simulink model "l17_ex1_LC"  (R2018b)
settings: Solver=ode45  StartTime=0.0  StopTime=5  MaxStep=1e-5  RelTol=1e-4  AbsTol=1e-4  EnableMultiTasking=on
values from neighbouring files (symbols this model uses):
  K = 1    [l16.m]    (also in l17.m = 5.3)
  p1 = 2.65    [l17.m]
  z1 = 1    [l17.m]
settings Model: Creator=Joe  LastModifiedBy=joema
settings SolverCC: AutoScaleAbsTol=off
settings DataIOCC: LimitDataPoints=on  SaveFormat=Array
settings OptimizationCC: LifeSpan=inf
settings DebuggingCC: UnderspecifiedInitializationDetection=Classic  MergeDetectMultiDrivingBlocksExec=none  LibraryContextMissingDiagnostic=none  SFUnexpectedBacktrackingDiag=warning  SFNoUnconditionalDefaultTransitionDiag=warning  SFExecutionAtInitializationDiag=none
settings HardwareCC: ProdBitPerPointer=32  ProdBitPerSizeT=32  ProdBitPerPtrDiffT=32  ProdLargestAtomicFloat=None  ProdIntDivRoundTo=Undefined  ProdEndianess=Unspecified  ProdWordSize=32  ProdHWDeviceType=32-bit Generic
settings ModelReferenceCC: PropagateSignalLabelsOutOfModel=off
settings SFSimCC: SimUseLocalCustomCode=off
settings RTWCC: RTWUseLocalCustomCode=off
settings CodeAppCC: StateflowObjectComments=on
settings GRTTargetCC: TargetLangStandard=C89/C90 (ANSI)  GeneratePreprocessorConditionals=Disable all
settings ConfigComp: CovMetricSettings=dw  CovHtmlReporting=on  CovSaveCumulativeToWorkspaceVar=on  CovSaveSingleToWorkspaceVar=on  CovExternalEMLEnable=off  CovSFcnEnable=off

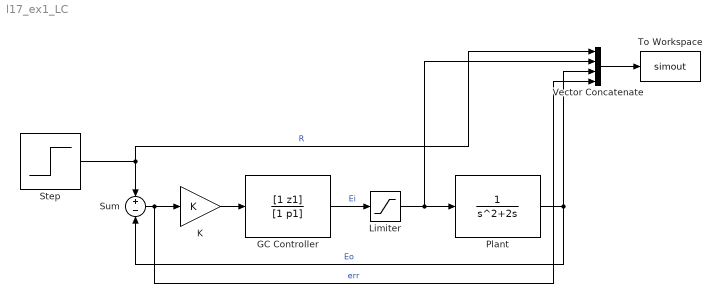
== system l17_ex1_LC ==
  GC Controller : TransferFcn  Numerator=[1 z1]  Denominator=[1 p1]
  K : Gain  Gain=K
  Limiter : Saturate  UpperLimit=1e2  LowerLimit=-1e2
  Plant : TransferFcn  Numerator=1  Denominator=[1 2 0]
  Step : Step  Time=0  After=5  SampleTime=0
  Sum : Sum  Inputs=+-
  To Workspace : ToWorkspace  VariableName=simout  SaveFormat=Timeseries  SampleTime=-1
  Vector Concatenate : Concatenate  NumInputs=4
  wires:
  Step/1 -> Sum/1, Vector Concatenate/1  "R"
  Sum/1 -> Vector Concatenate/4, K/1  "err"
  K/1 -> GC Controller/1
  Plant/1 -> Vector Concatenate/3, Sum/2  "Eo"
  Vector Concatenate/1 -> To Workspace/1
  GC Controller/1 -> Limiter/1  "Ei"
  Limiter/1 -> Vector Concatenate/2, Plant/1
